simulink model "AC_DC"  (R2022b)
settings: Solver=FixedStepDiscrete  StartTime=0.0  StopTime=2  FixedStep=1e-6  RelTol=1e-3
libraries: spsRMSLib x11, spsSeriesRLCBranchLib x9, simulink x7, spsVoltageMeasurementLib x7, spsCurrentMeasurementLib x6, spsMosfetLib x6, spsIdealSwitchLib x3, spsFourierLib x2, spsMeanLib x2, slpidlib x2, sps_lib x1, spsControlledVoltageSourceLib x1
(part 2 of 2)

== matlab function AC_DC/MATLAB Function22 ==
  data: alpha input; d output; beta input; theta input; q output
function [d, q] = Park_Transform(alpha, beta, theta)
% Park变换模块（直接输入SOGI-FLL的theta，无内部积分）
% 输入：
%   alpha - α轴分量（SOGI-FLL的U_prime）
%   beta  - β轴分量（SOGI-FLL的deltaU_prime）
%   theta - 瞬时相位（SOGI-FLL直接输出的theta）
% 输出：
%   d         - d轴（直轴）分量
%   q         - q轴（交轴）分量
%   cos_theta - 相位θ的余弦值（新增输出）
%   sin_theta - 相位θ的正弦值（新增输出）

%% 核心计算
cos_theta = cos(theta);  % 相位θ的余弦值
sin_theta = sin(theta);  % 相位θ的正弦值


% 修正后的 Park 变换公式（d轴对齐同相分量 beta）
d =  alpha * cos_theta + beta * sin_theta;
q = -alpha * sin_theta + beta * cos_theta;
end

== matlab function AC_DC/MATLAB Function16 ==
  data: in1 input; out1 output; in2 input; in3 input; in4 input; in5 input; in6 input; in7 input; t input; out2 output; out3 output; out4 output; out5 output; out6 output; out7 output
function [out1, out2, out3, out4, out5, out6, out7] = fcn(in1, in2, in3, in4, in5, in6, in7, t)
% 输入：
% in1~in7 : 7路采样信号
% t       : 仿真时间 (需连接Clock模块)
% 输出：
% out1~out7: 0.4秒前全为0，0.4秒后输出采样值

% ====================== 核心判断（只有一行） ======================
if t >= 0.4
    % 时间到：输出采样值
    out1 = in1;
    out2 = in2;
    out3 = in3;
    out4 = in4;
    out5 = in5;
    out6 = in6;
    out7 = in7;
else
    % 时间未到：全部输出0
    out1 = 0;
    out2 = 0;
    out3 = 0;
    out4 = 0;
    out5 = 0;
    out6 = 0;
    out7 = 0;
end

== matlab function AC_DC/MATLAB Function23 ==
  data: I_ref input; duty_out output; I_fb input
function duty_out = fcn(I_ref, I_fb)
%#codegen
% 同步Boost电流环PI控制器（带钳位抗饱和）
% 适配：20kHz采样、±5A电流传感器、占空比0.1~0.9安全范围
% 输入：
%   I_ref: 电压环输出的电流给定（对应你模型里电压环PI的输出）
%   I_fb: 电流反馈（对应你模型里经过-1增益后的IL信号）
% 输出：
%   duty_out: 最终占空比，直接接你模型里的1/z延迟模块

% 持久化变量：保存积分器状态，每个控制周期保留数值
persistent integral_val;
% 初始化：仅仿真启动的第一个控制周期执行1次
if isempty(integral_val)
    integral_val = 0;
end

% ==================== 1. 控制参数（和你原PI模块参数完全一致，可直接修改）====================
Kp = 0.5;       % 比例增益，和你原设置一致
Ki = 10;         % 积分增益，和你原设置一致
Ts = 5e-5;       % 20kHz控制周期，固定不变
% ==================== 2. 物理极限设置（核心抗饱和阈值）====================
DUTY_MAX = 0.93;  % 占空比上限，避免上下管直通
DUTY_MIN = -0.07;  % 占空比下限，杜绝轻载反向电流
I_SAT_LIMIT = 10; % 电流传感器饱和阈值，接近±5A量程提前触发保护

% ==================== 3. 误差计算 ====================
err = I_ref - I_fb;

% ==================== 4. 比例项输出 ====================
prop_out = Kp * err;

% ==================== 5. 核心抗饱和逻辑 ====================
% 5.1 积分项预计算
integral_inc = Ki * Ts * err;
integral_pre = integral_val + integral_inc;
% 5.2 预计算不饱和的PI输出
duty_pre = prop_out + integral_pre;

% 5.3 钳位抗饱和规则：
% 仅当输出在线性区、且电流未达到传感器饱和阈值时，才允许积分累加
% 同时加入反向积分放行规则，避免积分锁死
is_duty_linear = (duty_pre < DUTY_MAX) && (duty_pre > DUTY_MIN);
is_current_unsat = (abs(I_fb) < I_SAT_LIMIT);
is_integral_allow = is_duty_linear && is_current_unsat;
is_reverse_integral = (err > 0 && integral_pre < 0) || (err < 0 && integral_pre > 0);

if is_integral_allow || is_reverse_integral
    integral_val = integral_pre;
end

% ==================== 6. 最终占空比计算 + 硬限幅兜底 ====================
duty_out = prop_out + integral_val;
duty_out = min(max(duty_out, DUTY_MIN), DUTY_MAX);

== matlab function AC_DC/MATLAB Function24 ==
  settings: updateMethod=DISCRETE
  data: uin input; alpha output; beta output
function [alpha, beta] = SOGI_FLL_20kHz(uin)
% 严格对应你的 m 文件：20kHz 双线性 PI-FLL
% 输入：uin   单相电压
% 输出：alpha 同相输出 uα = x2
%      beta  正交输出 uβ = omega0*x3

%% 固定参数（和你的m文件完全一致）
dt = 5e-5;
K  = 1.414;
K1 = 0.25;
gamma_p =30;
gamma_i =500;
w_max = 2*pi*60;
w_min = 2*pi*40;

%% 状态持久化
persistent x1_prev x2_prev x3_prev omega0_prev U_prev integral_f first_run;
if isempty(first_run)
    x1_prev = 0;
    x2_prev = 0;
    x3_prev = 0;
    omega0_prev = 2*pi*50;
    U_prev = uin;
    integral_f = 0;
    first_run = false;
end

%% 1. 当前输入
U_curr = uin;
omega0_prev_local = omega0_prev;

%% 2. 频率预畸变
omega_pre = (2/dt) * tan(omega0_prev_local * dt / 2);

%% 3. 状态矩阵 A, B
A_mat = [
    -K1*omega_pre, -K1*omega_pre, 0;
    -K*omega_pre,  -K*omega_pre,  -omega_pre^2;
    0,              1,              0
];
B_mat = [
    K1*omega_pre;
    K*omega_pre;
    0
];

%% 4. 双线性变换
I_mat = eye(3);
M1 = I_mat - (dt/2)*A_mat;
M2 = I_mat + (dt/2)*A_mat;
U_avg = U_curr + U_prev;

x_prev_vec = [x1_prev; x2_prev; x3_prev];
x_curr_vec = M1 \ (M2 * x_prev_vec + (dt/2)*B_mat * U_avg);

x1_curr = x_curr_vec(1);
x2_curr = x_curr_vec(2);
x3_curr = x_curr_vec(3);

%% 5. PI-FLL 频率环
deltaU = U_curr - x1_curr - x2_curr;
deltaU_prime_val = omega0_prev_local * x3_curr;
epsilon_f = deltaU * deltaU_prime_val;

integral_f = integral_f + epsilon_f * dt;
domega0dt = -gamma_p * epsilon_f - gamma_i * integral_f;
omega0_curr = omega0_prev_local + dt * domega0dt;

% 频率限幅
omega0_curr = max(min(omega0_curr, w_max), w_min);

%% 6. 输出 alpha beta
alpha = x2_curr;
beta  = omega0_curr * x3_curr;

%% 7. 更新状态
x1_prev = x1_curr;
x2_prev = x2_curr;
x3_prev = x3_curr;
omega0_prev = omega0_curr;
U_prev = U_curr;

end

== matlab function AC_DC/MATLAB Function25 ==
  data: u_alpha input; theta output; u_beta input; qerror output
function [theta, qerror] = SRF_PLL(u_alpha, u_beta)
% 同步旋转坐标系锁相环 SRF-PLL
% 【已修改为：纯自适应频率版本 → 和你主循环PLL完全一致】
% 输入：u_alpha, u_beta
% 输出：theta 锁相相位, qerror q分量（趋近0）

    %% ===================== 1. 固定参数 =====================
    Ts = 5e-5;               % 20kHz 采样步长（必须匹配）
    
    % PI参数（和你主循环一致）
    kp_pll = 200;
    ki_pll = 7000;

    %% ===================== 2. 持久变量 =====================
    persistent theta_prev
    persistent integral_pll
    
    if isempty(theta_prev)
        theta_prev = 0;
        integral_pll = 0;
    end

    %% ===================== 3. Park 变换 =====================
    cos_theta = cos(theta_prev);
    sin_theta = sin(theta_prev);
    
    u_d =  u_alpha * cos_theta + u_beta * sin_theta;
    u_q = -u_alpha * sin_theta + u_beta * cos_theta;
    
    qerror = u_q;  % q分量（锁相成功→0）

    %% ===================== 4. PI控制器（我的版本：直接输出ω） =====================
    integral_pll = integral_pll + qerror * Ts;          % 积分
    omega_pll    = kp_pll * qerror + ki_pll * integral_pll; % 直接输出角频率

    %% ===================== 5. 积分生成相位 =====================
    theta = theta_prev + omega_pll * Ts;

    %% ===================== 6. 相位归一化（±π） =====================
    if theta > pi
        theta = theta - 2*pi;
    elseif theta < -pi
        theta = theta + 2*pi;
    end

    %% ===================== 7. 更新状态 =====================
    theta_prev = theta;
end

== matlab function AC_DC/MATLAB Function26 ==
  data: in1 input; in2 input; t input; y output
function y = fcn(in1, in2, t)
% 输入：
% in1：0.4秒 ~ 1.4秒 之间输出的信号
% in2：0.4秒前输出的信号
% t   ：仿真时间 (需连接Clock模块)
% 输出：
% y：三段式输出
%    t < 0.4s    → 输出 in2
%    0.4s ≤ t < 1.4s → 输出 in1
%    t ≥ 1.4s    → 输出 0

% ====================== 核心三段式时间判断 ======================
if t >= 1.4
    % 第三段：1.4秒及以后，强制输出0
    y = in1;
elseif t >= 0.4
    % 第二段：0.4秒到1.4秒之间，输出信号1 (in1)
    y = in1;
else
    % 第一段：0.4秒之前，输出信号2 (in2)
    y = in2;
end

== matlab function AC_DC/MATLAB Function15 ==
  data: IGm_total input; Igm_clean output
function Igm_clean = Notch_100Hz_IGm(IGm_total)
% 100Hz陷波滤波器，放在IGm求和后，滤除二次纹波
% 陷波频率100Hz，带宽6Hz，采样率20kHz
% 输入：IGm_total = IGm1 + IGm2
% 输出：Igm_clean = 滤除100Hz纹波后的纯直流信号

%% 历史变量
persistent x_prev1 x_prev2 y_prev1 y_prev2;

%% 固定参数
Ts = 1/20000;
f0 = 100;          % 陷波频率100Hz
bw = 6;            % 陷波带宽6Hz
w0 = 2*pi*f0;
wb = 2*pi*bw;

%% 双线性变换离散化系数
k = 2/Ts;
a0 = k^2 + wb*k + w0^2;
a1 = 2*(w0^2 - k^2);
a2 = k^2 - wb*k + w0^2;
b0 = k^2 + w0^2;
b1 = 2*(w0^2 - k^2);
b2 = k^2 + w0^2;

%% 归一化
b0 = b0/a0;
b1 = b1/a0;
b2 = b2/a0;
a1 = a1/a0;
a2 = a2/a0;

%% 初始化
if isempty(x_prev1)
    x_prev1 = 0; x_prev2 = 0;
    y_prev1 = 0; y_prev2 = 0;
end

%% 差分方程
Igm_clean = b0*IGm_total + b1*x_prev1 + b2*x_prev2 - a1*y_prev1 - a2*y_prev2;

%% 更新历史变量
x_prev2 = x_prev1;
x_prev1 = IGm_total;
y_prev2 = y_prev1;
y_prev1 = Igm_clean;

end

== matlab function AC_DC/MATLAB Function27 ==
  data: t input; utarget output
function utarget = fcn(t)
% 逻辑：
% 0~0.4s   输出 0
% 0.4~0.7s 从 43 平滑上升到 55（柔和曲线，无冲击）
% 0.7s后   保持 55

START_TIME = 0.4;
END_TIME   = 0.7;
INITIAL_V  = 45;
FINAL_V    = 55;

if t < START_TIME
    utarget = 0;                        % 0~0.4s 输出0
elseif t <= END_TIME
    % 平滑上升：余弦曲线（开始慢、中间快、收尾稳）
    tau = (t - START_TIME) / (END_TIME - START_TIME);
    tau_smooth = 0.5 * (1 - cos(pi * tau));  % 平滑曲线
    utarget = INITIAL_V + (FINAL_V - INITIAL_V) * tau_smooth;
else
    utarget = FINAL_V;                  % 0.7s后保持恒定
end

== matlab function AC_DC/MATLAB Function10 ==
  data: alpha input; d output; beta input; theta input; q output
function [d, q] = Park_Transform(alpha, beta, theta)
% Park变换模块（直接输入SOGI-FLL的theta，无内部积分）
% 输入：
%   alpha - α轴分量（SOGI-FLL的U_prime）
%   beta  - β轴分量（SOGI-FLL的deltaU_prime）
%   theta - 瞬时相位（SOGI-FLL直接输出的theta）
% 输出：
%   d         - d轴（直轴）分量
%   q         - q轴（交轴）分量
%   cos_theta - 相位θ的余弦值（新增输出）
%   sin_theta - 相位θ的正弦值（新增输出）

%% 核心计算
cos_theta = cos(theta);  % 相位θ的余弦值
sin_theta = sin(theta);  % 相位θ的正弦值


% 修正后的 Park 变换公式（d轴对齐同相分量 beta）
d =  alpha * cos_theta + beta * sin_theta;
q = -alpha * sin_theta + beta * cos_theta;
end

== matlab function AC_DC/MATLAB Function19 ==
  settings: updateMethod=DISCRETE
  data: uin input; alpha output; beta output
function [alpha, beta] = SOGI_FLL_20kHz(uin)
% 严格对应你的 m 文件：20kHz 双线性 PI-FLL
% 输入：uin   单相电压
% 输出：alpha 同相输出 uα = x2
%      beta  正交输出 uβ = omega0*x3

%% 固定参数（和你的m文件完全一致）
dt = 5e-5;
K  = 1.414;
K1 = 0.25;
gamma_p =30;
gamma_i =500;
w_max = 2*pi*60;
w_min = 2*pi*40;

%% 状态持久化
persistent x1_prev x2_prev x3_prev omega0_prev U_prev integral_f first_run;
if isempty(first_run)
    x1_prev = 0;
    x2_prev = 0;
    x3_prev = 0;
    omega0_prev = 2*pi*50;
    U_prev = uin;
    integral_f = 0;
    first_run = false;
end

%% 1. 当前输入
U_curr = uin;
omega0_prev_local = omega0_prev;

%% 2. 频率预畸变
omega_pre = (2/dt) * tan(omega0_prev_local * dt / 2);

%% 3. 状态矩阵 A, B
A_mat = [
    -K1*omega_pre, -K1*omega_pre, 0;
    -K*omega_pre,  -K*omega_pre,  -omega_pre^2;
    0,              1,              0
];
B_mat = [
    K1*omega_pre;
    K*omega_pre;
    0
];

%% 4. 双线性变换
I_mat = eye(3);
M1 = I_mat - (dt/2)*A_mat;
M2 = I_mat + (dt/2)*A_mat;
U_avg = U_curr + U_prev;

x_prev_vec = [x1_prev; x2_prev; x3_prev];
x_curr_vec = M1 \ (M2 * x_prev_vec + (dt/2)*B_mat * U_avg);

x1_curr = x_curr_vec(1);
x2_curr = x_curr_vec(2);
x3_curr = x_curr_vec(3);

%% 5. PI-FLL 频率环
deltaU = U_curr - x1_curr - x2_curr;
deltaU_prime_val = omega0_prev_local * x3_curr;
epsilon_f = deltaU * deltaU_prime_val;

integral_f = integral_f + epsilon_f * dt;
domega0dt = -gamma_p * epsilon_f - gamma_i * integral_f;
omega0_curr = omega0_prev_local + dt * domega0dt;

% 频率限幅
omega0_curr = max(min(omega0_curr, w_max), w_min);

%% 6. 输出 alpha beta
alpha = x2_curr;
beta  = omega0_curr * x3_curr;

%% 7. 更新状态
x1_prev = x1_curr;
x2_prev = x2_curr;
x3_prev = x3_curr;
omega0_prev = omega0_curr;
U_prev = U_curr;

end

== matlab function AC_DC/MATLAB Function2 ==
  data: u_alpha input; theta output; u_beta input; qerror output
function [theta, qerror] = SRF_PLL(u_alpha, u_beta)
% 同步旋转坐标系锁相环 SRF-PLL
% 【已修改为：纯自适应频率版本 → 和你主循环PLL完全一致】
% 输入：u_alpha, u_beta
% 输出：theta 锁相相位, qerror q分量（趋近0）

    %% ===================== 1. 固定参数 =====================
    Ts = 5e-5;               % 20kHz 采样步长（必须匹配）
    
    % PI参数（和你主循环一致）
    kp_pll = 200;
    ki_pll = 7000;

    %% ===================== 2. 持久变量 =====================
    persistent theta_prev
    persistent integral_pll
    
    if isempty(theta_prev)
        theta_prev = 0;
        integral_pll = 0;
    end

    %% ===================== 3. Park 变换 =====================
    cos_theta = cos(theta_prev);
    sin_theta = sin(theta_prev);
    
    u_d =  u_alpha * cos_theta + u_beta * sin_theta;
    u_q = -u_alpha * sin_theta + u_beta * cos_theta;
    
    qerror = u_q;  % q分量（锁相成功→0）

    %% ===================== 4. PI控制器（我的版本：直接输出ω） =====================
    integral_pll = integral_pll + qerror * Ts;          % 积分
    omega_pll    = kp_pll * qerror + ki_pll * integral_pll; % 直接输出角频率

    %% ===================== 5. 积分生成相位 =====================
    theta = theta_prev + omega_pll * Ts;

    %% ===================== 6. 相位归一化（±π） =====================
    if theta > pi
        theta = theta - 2*pi;
    elseif theta < -pi
        theta = theta + 2*pi;
    end

    %% ===================== 7. 更新状态 =====================
    theta_prev = theta;
end

== matlab function AC_DC/级联谐波抑制4 ==
  data: u input; y output
function y = Cascade_Notch_Filter(u)
% 级联陷波滤波器：滤除3/5/7次固定频率谐波（150/250/350Hz）
% 输入u：待滤波的标量信号
% 输出y：滤波后的标量信号
% 适配：20kHz采样率（Ts=5e-5），和你的控制环完全对齐

    persistent x3_1 x3_2 x5_1 x5_2 x7_1 x7_2 first_run
    persistent b3_0 b3_1 b3_2 a3_1 a3_2
    persistent b5_0 b5_1 b5_2 a5_1 a5_2
    persistent b7_0 b7_1 b7_2 a7_1 a7_2

    %% ===================== 1. 初始化：仅首次运行 =====================
    if isempty(first_run)
        % --- 固定参数 ---
        Fs = 2e4;          % 采样频率 20kHz
        Ts = 1/Fs;            % 采样周期 5e-5s
        wc = 10;              % 截止角频率 25 rad/s
        
        % 目标谐波频率
        w3 = 2*pi*150;  % 3次谐波 150Hz
        w5 = 2*pi*250;  % 5次谐波 250Hz
        w7 = 2*pi*350;  % 7次谐波 350Hz

        % --- Tustin变换预计算系数 ---
        k = 2/Ts;
        k2 = k*k;

        % --- 3次滤波器系数 ---
        [b3_0, b3_1, b3_2, a3_1, a3_2] = calc_coeff(w3, wc, k, k2);
        % --- 5次滤波器系数 ---
        [b5_0, b5_1, b5_2, a5_1, a5_2] = calc_coeff(w5, wc, k, k2);
        % --- 7次滤波器系数 ---
        [b7_0, b7_1, b7_2, a7_1, a7_2] = calc_coeff(w7, wc, k, k2);

        % --- 显式初始化状态变量为标量 ---
        x3_1 = 0; x3_2 = 0;
        x5_1 = 0; x5_2 = 0;
        x7_1 = 0; x7_2 = 0;
        
        first_run = 1;
    end

    %% ===================== 2. 级联滤波计算（显式差分方程） =====================
    % --- 第1级：3次谐波滤波 ---
    y3 = b3_0*u + x3_1;
    x3_1_next = b3_1*u - a3_1*y3 + x3_2;
    x3_2_next = b3_2*u - a3_2*y3;
    
    % --- 第2级：5次谐波滤波 ---
    y5 = b5_0*y3 + x5_1;
    x5_1_next = b5_1*y3 - a5_1*y5 + x5_2;
    x5_2_next = b5_2*y3 - a5_2*y5;
    
    % --- 第3级：7次谐波滤波 ---
    y7 = b7_0*y5 + x7_1;
    x7_1_next = b7_1*y5 - a7_1*y7 + x7_2;
    x7_2_next = b7_2*y5 - a7_2*y7;
    
    % --- 更新状态变量 ---
    x3_1 = x3_1_next; x3_2 = x3_2_next;
    x5_1 = x5_1_next; x5_2 = x5_2_next;
    x7_1 = x7_1_next; x7_2 = x7_2_next;
    
    % --- 最终输出 ---
    y = y7;

end

%% ===================== 局部函数：预计算滤波器系数 =====================
function [b0, b1, b2, a1, a2] = calc_coeff(wn, wc, k, k2)
    % 连续域：G(s) = (s^2 + wn^2) / (s^2 + 2*wc*s + wn^2)
    % Tustin离散化：s = k*(z-1)/(z+1)
    
    % 连续域系数
    num_b0 = 1; num_b1 = 0; num_b2 = wn^2;
    den_a0 = 1; den_a1 = 2*wc; den_a2 = wn^2;
    
    % 离散化计算
    B0 = num_b0*k2 + num_b1*k + num_b2;
    B1 = 2*num_b2 - 2*num_b0*k2;
    B2 = num_b0*k2 - num_b1*k + num_b2;
    
    A0 = den_a0*k2 + den_a1*k + den_a2;
    A1 = 2*den_a2 - 2*den_a0*k2;
    A2 = den_a0*k2 - den_a1*k + den_a2;
    
    % 归一化（a0=1）
    b0 = B0 / A0;
    b1 = B1 / A0;
    b2 = B2 / A0;
    a1 = A1 / A0;
    a2 = A2 / A0;
end

== matlab function AC_DC/MATLAB Function20 ==
  data: i_error input; m output
function m  = QPR_Current_Loop(i_error)
% 单相LCL整流器 电流环 多谐振QPR控制器
% 【严格匹配论文公式】G = Kp + Σ(2Kr·wi·s)/(s²+2wi·s + wn²)
% 谐振项：基波50Hz + 3次150Hz +5次250Hz +7次350Hz
% 【参数规则】仅Kp全局共用，Kr/wi/w0 每项独立设置
% 采样率：20kHz | 双线性变换离散化

%% ===================== 独立历史变量 =====================
persistent e1_1 e1_2 m1_1 m1_2  % 基波 n=1
persistent e3_1 e3_2 m3_1 m3_2  % 3次  n=3
persistent e5_1 e5_2 m5_1 m5_2  % 5次  n=5
persistent e7_1 e7_2 m7_1 m7_2  % 7次  n=7

%% ===================== 全局共用参数（仅Kp） =====================
Ts    = 1/20000;   % 采样周期
Kp    =0.3;       % 【唯一共用参数】比例增益

%% ===================== 各谐振项 独立参数（互不共用） =====================
% === 基波 50Hz (n=1) ===
Kr1 = 40;
wi1 = 10;
w01 = 100*pi;

% === 3次谐波 150Hz (n=3) ===
Kr3 = 100;
wi3 = 6;
w03 = 300*pi;

% === 5次谐波 250Hz (n=5) ===
Kr5 = 80;
wi5 = 6;
w05 = 500*pi;

% === 7次谐波 350Hz (n=7) ===
Kr7 = 60;
wi7 = 6;
w07 = 700*pi;

%% ===================== 初始化 =====================
if isempty(e1_1)
    e1_1=0;e1_2=0;m1_1=0;m1_2=0;
    e3_1=0;e3_2=0;m3_1=0;m3_2=0;
    e5_1=0;e5_2=0;m5_1=0;m5_2=0;
    e7_1=0;e7_2=0;m7_1=0;m7_2=0;
end

%% ===================== 1. 共用比例项 =====================
m_p = Kp * i_error;

%% ===================== 2. 基波谐振项计算 =====================
A1  = 2 * Kr1 * wi1;
B1  = 2 * wi1;
C1  = w01^2;
a0_1 = 4 + 2*B1*Ts + C1*Ts^2;
a1_1 = -8 + 2*C1*Ts^2;
a2_1 = 4 - 2*B1*Ts + C1*Ts^2;
b0_1 =  A1 * Ts;
b1_1 =  0;
b2_1 = -A1 * Ts;
m1 = (b0_1*i_error + b1_1*e1_1 + b2_1*e1_2 - a1_1*m1_1 - a2_1*m1_2) / a0_1;
% 更新
e1_2 = e1_1; e1_1 = i_error;
m1_2 = m1_1; m1_1 = m1;

%% ===================== 3. 3次谐波谐振项计算 =====================
A3  = 2 * Kr3 * wi3;
B3  = 2 * wi3;
C3  = w03^2;
a0_3 = 4 + 2*B3*Ts + C3*Ts^2;
a1_3 = -8 + 2*C3*Ts^2;
a2_3 = 4 - 2*B3*Ts + C3*Ts^2;
b0_3 =  A3 * Ts;
b1_3 =  0;
b2_3 = -A3 * Ts;
m3 = (b0_3*i_error + b1_3*e3_1 + b2_3*e3_2 - a1_3*m3_1 - a2_3*m3_2) / a0_3;
% 更新
e3_2 = e3_1; e3_1 = i_error;
m3_2 = m3_1; m3_1 = m3;

%% ===================== 4. 5次谐波谐振项计算 =====================
A5  = 2 * Kr5 * wi5;
B5  = 2 * wi5;
C5  = w05^2;
a0_5 = 4 + 2*B5*Ts + C5*Ts^2;
a1_5 = -8 + 2*C5*Ts^2;
a2_5 = 4 - 2*B5*Ts + C5*Ts^2;
b0_5 =  A5 * Ts;
b1_5 =  0;
b2_5 = -A5 * Ts;
m5 = (b0_5*i_error + b1_5*e5_1 + b2_5*e5_2 - a1_5*m5_1 - a2_5*m5_2) / a0_5;
% 更新
e5_2 = e5_1; e5_1 = i_error;
m5_2 = m5_1; m5_1 = m5;

%% ===================== 5. 7次谐波谐振项计算 =====================
A7  = 2 * Kr7 * wi7;
B7  = 2 * wi7;
C7  = w07^2;
a0_7 = 4 + 2*B7*Ts + C7*Ts^2;
a1_7 = -8 + 2*C7*Ts^2;
a2_7 = 4 - 2*B7*Ts + C7*Ts^2;
b0_7 =  A7 * Ts;
b1_7 =  0;
b2_7 = -A7 * Ts;
m7 = (b0_7*i_error + b1_7*e7_1 + b2_7*e7_2 - a1_7*m7_1 - a2_7*m7_2) / a0_7;
% 更新
e7_2 = e7_1; e7_1 = i_error;
m7_2 = m7_1; m7_1 = m7;

%% ===================== 总输出叠加 =====================
m = m_p + m1 + m3 + m5 + m7;



end

== matlab function AC_DC/合闸后再传入信号1 ==
  data: t input; Uref output; Udc input; Udc_error output
function [Uref, Udc_error] = Udc_Control_Logic(t, Udc)
% 单相整流器 直流母线电压 合闸综合控制逻辑
% 功能：
%   1. 0.15s合闸前：Uref=0，不计算误差（Udc_error=0）
%   2. 0.15s后：Uref直接跳变到40V，开始计算误差 Udc_error = 40 - Udc
% 输入：
%   t: 仿真时间
%   Udc: 实际直流母线电压测量值
% 输出：
%   Uref: 直流母线电压给定值
%   Udc_error: 电压误差 = Uref - Udc（合闸后才有值）

persistent V_target t_start;
if isempty(V_target)
    V_target =55;      % 目标电压，直接给50V
    t_start = 0.15;     % 合闸时间
end

%% 核心逻辑：时间分段控制
if t < t_start
    % === 阶段1：合闸前 ===
    Uref = 0;           % 电压给定为0
    Udc_error = 0;      % 不计算误差，避免误动作
else
    % === 阶段2：合闸后 ===
    Uref = V_target;    % 直接跳变到40V恒定
    Udc_error = Uref - Udc; % 立刻开始计算误差，投入闭环
end

end

== matlab function AC_DC/模仿开关控制3 ==
  data: t input; mod_out output; mod_in input
function mod_out = gate_mod_signal(t, mod_in)
% 功能：0.25s前输出0，0.25s后输出原调制波mod_in
% 输入 t: 仿真时间 (Clock模块)
% 输入 mod_in: 原始调制波信号
% 输出 mod_out: 带使能的调制波信号

t_start =0.15; % 合闸时间

if t < t_start
    mod_out = 0;          % 合闸前强制输出0
else
    mod_out = mod_in;      % 合闸后输出原调制波
end
end

== matlab function AC_DC/MATLAB Function28 ==
  data: in1 input; in2 input; t input; y output
function y = fcn(in1, in2, t)
% 输入：
% in1：0.4秒 ~ 1.4秒 之间输出的信号
% in2：0.4秒前输出的信号
% t   ：仿真时间 (需连接Clock模块)
% 输出：
% y：三段式输出
%    t < 0.4s    → 输出 in2
%    0.4s ≤ t < 1.4s → 输出 in1
%    t ≥ 1.4s    → 输出 0

% ====================== 核心三段式时间判断 ======================
if t >= 1.7
    % 第三段：1.4秒及以后，强制输出0
    y = in2;
elseif t >= 0.4
    % 第二段：0.4秒到1.4秒之间，输出信号1 (in1)
    y = in1;
else
    % 第一段：0.4秒之前，输出信号2 (in2)
    y = in1;
end

== matlab function AC_DC/级联谐波抑制2 ==
  data: u input; y output
function y = Cascade_Notch_Filter(u)
% 级联陷波滤波器：滤除3/5/7次固定频率谐波（150/250/350Hz）
% 输入u：待滤波的标量信号
% 输出y：滤波后的标量信号
% 适配：20kHz采样率（Ts=5e-5），和你的控制环完全对齐

    persistent x3_1 x3_2 x5_1 x5_2 x7_1 x7_2 first_run
    persistent b3_0 b3_1 b3_2 a3_1 a3_2
    persistent b5_0 b5_1 b5_2 a5_1 a5_2
    persistent b7_0 b7_1 b7_2 a7_1 a7_2

    %% ===================== 1. 初始化：仅首次运行 =====================
    if isempty(first_run)
        % --- 固定参数 ---
        Fs = 2e4;          % 采样频率 20kHz
        Ts = 1/Fs;            % 采样周期 5e-5s
        wc = 10;              % 截止角频率 25 rad/s
        
        % 目标谐波频率
        w3 = 2*pi*150;  % 3次谐波 150Hz
        w5 = 2*pi*250;  % 5次谐波 250Hz
        w7 = 2*pi*350;  % 7次谐波 350Hz

        % --- Tustin变换预计算系数 ---
        k = 2/Ts;
        k2 = k*k;

        % --- 3次滤波器系数 ---
        [b3_0, b3_1, b3_2, a3_1, a3_2] = calc_coeff(w3, wc, k, k2);
        % --- 5次滤波器系数 ---
        [b5_0, b5_1, b5_2, a5_1, a5_2] = calc_coeff(w5, wc, k, k2);
        % --- 7次滤波器系数 ---
        [b7_0, b7_1, b7_2, a7_1, a7_2] = calc_coeff(w7, wc, k, k2);

        % --- 显式初始化状态变量为标量 ---
        x3_1 = 0; x3_2 = 0;
        x5_1 = 0; x5_2 = 0;
        x7_1 = 0; x7_2 = 0;
        
        first_run = 1;
    end

    %% ===================== 2. 级联滤波计算（显式差分方程） =====================
    % --- 第1级：3次谐波滤波 ---
    y3 = b3_0*u + x3_1;
    x3_1_next = b3_1*u - a3_1*y3 + x3_2;
    x3_2_next = b3_2*u - a3_2*y3;
    
    % --- 第2级：5次谐波滤波 ---
    y5 = b5_0*y3 + x5_1;
    x5_1_next = b5_1*y3 - a5_1*y5 + x5_2;
    x5_2_next = b5_2*y3 - a5_2*y5;
    
    % --- 第3级：7次谐波滤波 ---
    y7 = b7_0*y5 + x7_1;
    x7_1_next = b7_1*y5 - a7_1*y7 + x7_2;
    x7_2_next = b7_2*y5 - a7_2*y7;
    
    % --- 更新状态变量 ---
    x3_1 = x3_1_next; x3_2 = x3_2_next;
    x5_1 = x5_1_next; x5_2 = x5_2_next;
    x7_1 = x7_1_next; x7_2 = x7_2_next;
    
    % --- 最终输出 ---
    y = y7;

end

%% ===================== 局部函数：预计算滤波器系数 =====================
function [b0, b1, b2, a1, a2] = calc_coeff(wn, wc, k, k2)
    % 连续域：G(s) = (s^2 + wn^2) / (s^2 + 2*wc*s + wn^2)
    % Tustin离散化：s = k*(z-1)/(z+1)
    
    % 连续域系数
    num_b0 = 1; num_b1 = 0; num_b2 = wn^2;
    den_a0 = 1; den_a1 = 2*wc; den_a2 = wn^2;
    
    % 离散化计算
    B0 = num_b0*k2 + num_b1*k + num_b2;
    B1 = 2*num_b2 - 2*num_b0*k2;
    B2 = num_b0*k2 - num_b1*k + num_b2;
    
    A0 = den_a0*k2 + den_a1*k + den_a2;
    A1 = 2*den_a2 - 2*den_a0*k2;
    A2 = den_a0*k2 - den_a1*k + den_a2;
    
    % 归一化（a0=1）
    b0 = B0 / A0;
    b1 = B1 / A0;
    b2 = B2 / A0;
    a1 = A1 / A0;
    a2 = A2 / A0;
end

== matlab function AC_DC/MATLAB Function29 ==
  data: i_error input; m output
% function m  = QPR_Current_Loop(i_error, t)
% %#codegen
% % 单相LCL整流器 电流环 多谐振QPR控制器【仅动态调整Kp】
% % 动态Kp规则：
% %   t < 0.4s：Kp=0.3（保持原值，开环前不工作）
% %   0.4s ≤ t < 1.0s：Kp从10线性平滑降到0.3（延长下降时间）
% %   t ≥ 1.0s：Kp=0.3（稳态小Kp，不放大纹波）
% % 其他谐振项计算完全保留你原有的逻辑
% 
% %% ===================== 独立历史变量 =====================
% persistent e1_1 e1_2 m1_1 m1_2  % 基波 n=1
% persistent e3_1 e3_2 m3_1 m3_2  % 3次  n=3
% persistent e5_1 e5_2 m5_1 m5_2  % 5次  n=5
% persistent e7_1 e7_2 m7_1 m7_2  % 7次  n=7
% 
% %% ===================== 全局共用参数 =====================
% Ts    = 1/20000;   % 采样周期
% 
% %% ===================== 各谐振项 独立参数（完全保留你的原值）=====================
% % === 基波 50Hz (n=1) ===
% Kr1 = 40;
% wi1 = 6;
% w01 = 100*pi;
% 
% % === 3次谐波 150Hz (n=3) ===
% Kr3 = 100;
% wi3 = 6;
% w03 = 300*pi;
% 
% % === 5次谐波 250Hz (n=5) ===
% Kr5 = 80;
% wi5 = 6;
% w05 = 500*pi;
% 
% % === 7次谐波 350Hz (n=7) ===
% Kr7 = 60;
% wi7 = 6;
% w07 = 700*pi;
% 
% %% ===================== 初始化 =====================
% if isempty(e1_1)
%     e1_1=0;e1_2=0;m1_1=0;m1_2=0;
%     e3_1=0;e3_2=0;m3_1=0;m3_2=0;
%     e5_1=0;e5_2=0;m5_1=0;m5_2=0;
%     e7_1=0;e7_2=0;m7_1=0;m7_2=0;
% end
% 
% %% ===================== 核心：仅动态调整Kp（平滑曲线版本） =====================
% t_start = 0.4;  % 开环时间
% t_end   = 1;  % 结束时间
% Kp_start = 0.3;  % 起始值
% Kp_end   = 0.3; % 最终稳态值
% 
% if t < t_start
%     Kp = 0.3;
% elseif t >= t_start && t < t_end
%     % 归一化时间 0~1
%     tau = (t - t_start) / (t_end - t_start);
%     % 余弦平滑曲线：开始慢、中间快、结束慢 → 无超调无冲击
%     tau_smooth = 0.5 * (1 - cos(pi * tau));
%     % 计算平滑Kp
%     Kp = Kp_start - (Kp_start - Kp_end) * tau_smooth;
% else
%     Kp = Kp_end;
% end
% %% ===================== 1. 共用比例项（用动态Kp）=====================
% 
% m_p = Kp * i_error;
% 
% %% ===================== 2. 基波谐振项计算（完全保留你的逻辑）=====================
% A1  = 2 * Kr1 * wi1;
% B1  = 2 * wi1;
% C1  = w01^2;
% a0_1 = 4 + 2*B1*Ts + C1*Ts^2;
% a1_1 = -8 + 2*C1*Ts^2;
% a2_1 = 4 - 2*B1*Ts + C1*Ts^2;
% b0_1 =  A1 * Ts;
% b1_1 =  0;
% b2_1 = -A1 * Ts;
% m1 = (b0_1*i_error + b1_1*e1_1 + b2_1*e1_2 - a1_1*m1_1 - a2_1*m1_2) / a0_1;
% % 更新
% e1_2 = e1_1; e1_1 = i_error;
% m1_2 = m1_1; m1_1 = m1;
% 
% %% ===================== 3. 3次谐波谐振项计算（完全保留你的逻辑）=====================
% A3  = 2 * Kr3 * wi3;
% B3  = 2 * wi3;
% C3  = w03^2;
% a0_3 = 4 + 2*B3*Ts + C3*Ts^2;
% a1_3 = -8 + 2*C3*Ts^2;
% a2_3 = 4 - 2*B3*Ts + C3*Ts^2;
% b0_3 =  A3 * Ts;
% b1_3 =  0;
% b2_3 = -A3 * Ts;
% m3 = (b0_3*i_error + b1_3*e3_1 + b2_3*e3_2 - a1_3*m3_1 - a2_3*m3_2) / a0_3;
% % 更新
% e3_2 = e3_1; e3_1 = i_error;
% m3_2 = m3_1; m3_1 = m3;
% 
% %% ===================== 4. 5次谐波谐振项计算（完全保留你的逻辑）=====================
% A5  = 2 * Kr5 * wi5;
% B5  = 2 * wi5;
% C5  = w05^2;
% a0_5 = 4 + 2*B5*Ts + C5*Ts^2;
% a1_5 = -8 + 2*C5*Ts^2;
% a2_5 = 4 - 2*B5*Ts + C5*Ts^2;
% b0_5 =  A5 * Ts;
% b1_5 =  0;
% b2_5 = -A5 * Ts;
% m5 = (b0_5*i_error + b1_5*e5_1 + b2_5*e5_2 - a1_5*m5_1 - a2_5*m5_2) / a0_5;
% % 更新
% e5_2 = e5_1; e5_1 = i_error;
% m5_2 = m5_1; m5_1 = m5;
% 
% %% ===================== 5. 7次谐波谐振项计算（完全保留你的逻辑）=====================
% A7  = 2 * Kr7 * wi7;
% B7  = 2 * wi7;
% C7  = w07^2;
% a0_7 = 4 + 2*B7*Ts + C7*Ts^2;
% a1_7 = -8 + 2*C7*Ts^2;
% a2_7 = 4 - 2*B7*Ts + C7*Ts^2;
% b0_7 =  A7 * Ts;
% b1_7 =  0;
% b2_7 = -A7 * Ts;
% m7 = (b0_7*i_error + b1_7*e7_1 + b2_7*e7_2 - a1_7*m7_1 - a2_7*m7_2) / a0_7;
% % 更新
% e7_2 = e7_1; e7_1 = i_error;
% m7_2 = m7_1; m7_1 = m7;
% 
% %% ===================== 总输出叠加 =====================
% m = m_p + m1 + m3 + m5 + m7;
% 
% end


function m  = QPR_Current_Loop(i_error)
%#codegen
% 单相LCL整流器 电流环 多谐振QPR控制器【固定Kp=0.3 + 频率预畸变】
% 特点：加入双线性变换频率预畸变，保证数字谐振频率准确

%% ===================== 独立历史变量 =====================
persistent e1_1 e1_2 m1_1 m1_2  % 基波 n=1
persistent e3_1 e3_2 m3_1 m3_2  % 3次  n=3
persistent e5_1 e5_2 m5_1 m5_2  % 5次  n=5
persistent e7_1 e7_2 m7_1 m7_2  % 7次  n=7

%% ===================== 全局共用参数 =====================
Ts    = 1/20000;   % 采样周期
Kp    = 0.3;        % 固定比例增益

%% ===================== 各谐振项 独立参数（含频率预畸变）=====================
% === 基波 50Hz (n=1) ===
Kr1 = 40;
wi1 = 6;
f1 = 50;
omega_analog_1 = 2*pi*f1;
w01 = (2/Ts)*tan(omega_analog_1*Ts/2); % 频率预畸变

% === 3次谐波 150Hz (n=3) ===
Kr3 = 100;
wi3 = 6;
f3 = 150;
omega_analog_3 = 2*pi*f3;
w03 = (2/Ts)*tan(omega_analog_3*Ts/2); % 频率预畸变

% === 5次谐波 250Hz (n=5) ===
Kr5 = 80;
wi5 = 6;
f5 = 250;
omega_analog_5 = 2*pi*f5;
w05 = (2/Ts)*tan(omega_analog_5*Ts/2); % 频率预畸变

% === 7次谐波 350Hz (n=7) ===
Kr7 = 60;
wi7 = 6;
f7 = 350;
omega_analog_7 = 2*pi*f7;
w07 = (2/Ts)*tan(omega_analog_7*Ts/2); % 频率预畸变

%% ===================== 初始化 =====================
if isempty(e1_1)
    e1_1=0;e1_2=0;m1_1=0;m1_2=0;
    e3_1=0;e3_2=0;m3_1=0;m3_2=0;
    e5_1=0;e5_2=0;m5_1=0;m5_2=0;
    e7_1=0;e7_2=0;m7_1=0;m7_2=0;
end

%% ===================== 1. 共用比例项（固定Kp）=====================
m_p = Kp * i_error;

%% ===================== 2. 基波谐振项计算 =====================
A1  = 2 * Kr1 * wi1;
B1  = 2 * wi1;
C1  = w01^2;
a0_1 = 4 + 2*B1*Ts + C1*Ts^2;
a1_1 = -8 + 2*C1*Ts^2;
a2_1 = 4 - 2*B1*Ts + C1*Ts^2;
b0_1 =  A1 * Ts;
b1_1 =  0;
b2_1 = -A1 * Ts;
m1 = (b0_1*i_error + b1_1*e1_1 + b2_1*e1_2 - a1_1*m1_1 - a2_1*m1_2) / a0_1;
% 更新
e1_2 = e1_1; e1_1 = i_error;
m1_2 = m1_1; m1_1 = m1;

%% ===================== 3. 3次谐波谐振项计算 =====================
A3  = 2 * Kr3 * wi3;
B3  = 2 * wi3;
C3  = w03^2;
a0_3 = 4 + 2*B3*Ts + C3*Ts^2;
a1_3 = -8 + 2*C3*Ts^2;
a2_3 = 4 - 2*B3*Ts + C3*Ts^2;
b0_3 =  A3 * Ts;
b1_3 =  0;
b2_3 = -A3 * Ts;
m3 = (b0_3*i_error + b1_3*e3_1 + b2_3*e3_2 - a1_3*m3_1 - a2_3*m3_2) / a0_3;
% 更新
e3_2 = e3_1; e3_1 = i_error;
m3_2 = m3_1; m3_1 = m3;

%% ===================== 4. 5次谐波谐振项计算 =====================
A5  = 2 * Kr5 * wi5;
B5  = 2 * wi5;
C5  = w05^2;
a0_5 = 4 + 2*B5*Ts + C5*Ts^2;
a1_5 = -8 + 2*C5*Ts^2;
a2_5 = 4 - 2*B5*Ts + C5*Ts^2;
b0_5 =  A5 * Ts;
b1_5 =  0;
b2_5 = -A5 * Ts;
m5 = (b0_5*i_error + b1_5*e5_1 + b2_5*e5_2 - a1_5*m5_1 - a2_5*m5_2) / a0_5;
% 更新
e5_2 = e5_1; e5_1 = i_error;
m5_2 = m5_1; m5_1 = m5;

%% ===================== 5. 7次谐波谐振项计算 =====================
A7  = 2 * Kr7 * wi7;
B7  = 2 * wi7;
C7  = w07^2;
a0_7 = 4 + 2*B7*Ts + C7*Ts^2;
a1_7 = -8 + 2*C7*Ts^2;
a2_7 = 4 - 2*B7*Ts + C7*Ts^2;
b0_7 =  A7 * Ts;
b1_7 =  0;
b2_7 = -A7 * Ts;
m7 = (b0_7*i_error + b1_7*e7_1 + b2_7*e7_2 - a1_7*m7_1 - a2_7*m7_2) / a0_7;
% 更新
e7_2 = e7_1; e7_1 = i_error;
m7_2 = m7_1; m7_1 = m7;

%% ===================== 总输出叠加 =====================
m = m_p + m1 + m3 + m5 + m7;

end

== matlab function AC_DC/MATLAB Function3 ==
  data: alpha input; d output; beta input; theta input; q output
function [d, q] = Park_Transform(alpha, beta, theta)
% Park变换模块（直接输入SOGI-FLL的theta，无内部积分）
% 输入：
%   alpha - α轴分量（SOGI-FLL的U_prime）
%   beta  - β轴分量（SOGI-FLL的deltaU_prime）
%   theta - 瞬时相位（SOGI-FLL直接输出的theta）
% 输出：
%   d         - d轴（直轴）分量
%   q         - q轴（交轴）分量
%   cos_theta - 相位θ的余弦值（新增输出）
%   sin_theta - 相位θ的正弦值（新增输出）

%% 核心计算
cos_theta = cos(theta);  % 相位θ的余弦值
sin_theta = sin(theta);  % 相位θ的正弦值


% 修正后的 Park 变换公式（d轴对齐同相分量 beta）
d =  alpha * cos_theta + beta * sin_theta;
q = -alpha * sin_theta + beta * cos_theta;
end

== matlab function AC_DC/MATLAB Function4 ==
  data: I_ref input; duty_out output; I_fb input
function duty_out = fcn(I_ref, I_fb)
%#codegen
% 同步Boost电流环PI控制器（带钳位抗饱和）
% 适配：20kHz采样、±5A电流传感器、占空比0.1~0.9安全范围
% 输入：
%   I_ref: 电压环输出的电流给定（对应你模型里电压环PI的输出）
%   I_fb: 电流反馈（对应你模型里经过-1增益后的IL信号）
% 输出：
%   duty_out: 最终占空比，直接接你模型里的1/z延迟模块

% 持久化变量：保存积分器状态，每个控制周期保留数值
persistent integral_val;
% 初始化：仅仿真启动的第一个控制周期执行1次
if isempty(integral_val)
    integral_val = 0;
end

% ==================== 1. 控制参数（和你原PI模块参数完全一致，可直接修改）====================
Kp = 0.5;       % 比例增益，和你原设置一致
Ki = 10;         % 积分增益，和你原设置一致
Ts = 5e-5;       % 20kHz控制周期，固定不变
% ==================== 2. 物理极限设置（核心抗饱和阈值）====================
DUTY_MAX = 0.93;  % 占空比上限，避免上下管直通
DUTY_MIN = -0.07;  % 占空比下限，杜绝轻载反向电流
I_SAT_LIMIT = 10; % 电流传感器饱和阈值，接近±5A量程提前触发保护

% ==================== 3. 误差计算 ====================
err = I_ref - I_fb;

% ==================== 4. 比例项输出 ====================
prop_out = Kp * err;

% ==================== 5. 核心抗饱和逻辑 ====================
% 5.1 积分项预计算
integral_inc = Ki * Ts * err;
integral_pre = integral_val + integral_inc;
% 5.2 预计算不饱和的PI输出
duty_pre = prop_out + integral_pre;

% 5.3 钳位抗饱和规则：
% 仅当输出在线性区、且电流未达到传感器饱和阈值时，才允许积分累加
% 同时加入反向积分放行规则，避免积分锁死
is_duty_linear = (duty_pre < DUTY_MAX) && (duty_pre > DUTY_MIN);
is_current_unsat = (abs(I_fb) < I_SAT_LIMIT);
is_integral_allow = is_duty_linear && is_current_unsat;
is_reverse_integral = (err > 0 && integral_pre < 0) || (err < 0 && integral_pre > 0);

if is_integral_allow || is_reverse_integral
    integral_val = integral_pre;
end

% ==================== 6. 最终占空比计算 + 硬限幅兜底 ====================
duty_out = prop_out + integral_val;
duty_out = min(max(duty_out, DUTY_MIN), DUTY_MAX);

== matlab function AC_DC/MATLAB Function5 ==
  settings: updateMethod=DISCRETE
  data: uin input; alpha output; beta output
function [alpha, beta] = SOGI_FLL_20kHz(uin)
% 严格对应你的 m 文件：20kHz 双线性 PI-FLL
% 输入：uin   单相电压
% 输出：alpha 同相输出 uα = x2
%      beta  正交输出 uβ = omega0*x3

%% 固定参数（和你的m文件完全一致）
dt = 5e-5;
K  = 1.414;
K1 = 0.25;
gamma_p =30;
gamma_i =500;
w_max = 2*pi*60;
w_min = 2*pi*40;

%% 状态持久化
persistent x1_prev x2_prev x3_prev omega0_prev U_prev integral_f first_run;
if isempty(first_run)
    x1_prev = 0;
    x2_prev = 0;
    x3_prev = 0;
    omega0_prev = 2*pi*50;
    U_prev = uin;
    integral_f = 0;
    first_run = false;
end

%% 1. 当前输入
U_curr = uin;
omega0_prev_local = omega0_prev;

%% 2. 频率预畸变
omega_pre = (2/dt) * tan(omega0_prev_local * dt / 2);

%% 3. 状态矩阵 A, B
A_mat = [
    -K1*omega_pre, -K1*omega_pre, 0;
    -K*omega_pre,  -K*omega_pre,  -omega_pre^2;
    0,              1,              0
];
B_mat = [
    K1*omega_pre;
    K*omega_pre;
    0
];

%% 4. 双线性变换
I_mat = eye(3);
M1 = I_mat - (dt/2)*A_mat;
M2 = I_mat + (dt/2)*A_mat;
U_avg = U_curr + U_prev;

x_prev_vec = [x1_prev; x2_prev; x3_prev];
x_curr_vec = M1 \ (M2 * x_prev_vec + (dt/2)*B_mat * U_avg);

x1_curr = x_curr_vec(1);
x2_curr = x_curr_vec(2);
x3_curr = x_curr_vec(3);

%% 5. PI-FLL 频率环
deltaU = U_curr - x1_curr - x2_curr;
deltaU_prime_val = omega0_prev_local * x3_curr;
epsilon_f = deltaU * deltaU_prime_val;

integral_f = integral_f + epsilon_f * dt;
domega0dt = -gamma_p * epsilon_f - gamma_i * integral_f;
omega0_curr = omega0_prev_local + dt * domega0dt;

% 频率限幅
omega0_curr = max(min(omega0_curr, w_max), w_min);

%% 6. 输出 alpha beta
alpha = x2_curr;
beta  = omega0_curr * x3_curr;

%% 7. 更新状态
x1_prev = x1_curr;
x2_prev = x2_curr;
x3_prev = x3_curr;
omega0_prev = omega0_curr;
U_prev = U_curr;

end

== matlab function AC_DC/MATLAB Function6 ==
  data: u_alpha input; theta output; u_beta input; qerror output
function [theta, qerror] = SRF_PLL(u_alpha, u_beta)
% 同步旋转坐标系锁相环 SRF-PLL
% 【已修改为：纯自适应频率版本 → 和你主循环PLL完全一致】
% 输入：u_alpha, u_beta
% 输出：theta 锁相相位, qerror q分量（趋近0）

    %% ===================== 1. 固定参数 =====================
    Ts = 5e-5;               % 20kHz 采样步长（必须匹配）
    
    % PI参数（和你主循环一致）
    kp_pll = 200;
    ki_pll = 7000;

    %% ===================== 2. 持久变量 =====================
    persistent theta_prev
    persistent integral_pll
    
    if isempty(theta_prev)
        theta_prev = 0;
        integral_pll = 0;
    end

    %% ===================== 3. Park 变换 =====================
    cos_theta = cos(theta_prev);
    sin_theta = sin(theta_prev);
    
    u_d =  u_alpha * cos_theta + u_beta * sin_theta;
    u_q = -u_alpha * sin_theta + u_beta * cos_theta;
    
    qerror = u_q;  % q分量（锁相成功→0）

    %% ===================== 4. PI控制器（我的版本：直接输出ω） =====================
    integral_pll = integral_pll + qerror * Ts;          % 积分
    omega_pll    = kp_pll * qerror + ki_pll * integral_pll; % 直接输出角频率

    %% ===================== 5. 积分生成相位 =====================
    theta = theta_prev + omega_pll * Ts;

    %% ===================== 6. 相位归一化（±π） =====================
    if theta > pi
        theta = theta - 2*pi;
    elseif theta < -pi
        theta = theta + 2*pi;
    end

    %% ===================== 7. 更新状态 =====================
    theta_prev = theta;
end

== matlab function AC_DC/MATLAB Function7 ==
  data: in1 input; in2 input; t input; y output
function y = fcn(in1, in2, t)
% 输入：
% in1：0.4秒 ~ 1.4秒 之间输出的信号
% in2：0.4秒前输出的信号
% t   ：仿真时间 (需连接Clock模块)
% 输出：
% y：三段式输出
%    t < 0.4s    → 输出 in2
%    0.4s ≤ t < 1.4s → 输出 in1
%    t ≥ 1.4s    → 输出 0

% ====================== 核心三段式时间判断 ======================
if t >= 1.4
    % 第三段：1.4秒及以后，强制输出0
    y = in1;
elseif t >= 0.4
    % 第二段：0.4秒到1.4秒之间，输出信号1 (in1)
    y = in1;
else
    % 第一段：0.4秒之前，输出信号2 (in2)
    y = in2;
end

== matlab function AC_DC/MATLAB Function8 ==
  data: t input; utarget output
function utarget = fcn(t)
% 逻辑：
% 0~0.4s   输出 0
% 0.4~0.7s 从 43 平滑上升到 55（柔和曲线，无冲击）
% 0.7s后   保持 55

START_TIME = 0.4;
END_TIME   = 0.7;
INITIAL_V  = 45;
FINAL_V    = 55;

if t < START_TIME
    utarget = 0;                        % 0~0.4s 输出0
elseif t <= END_TIME
    % 平滑上升：余弦曲线（开始慢、中间快、收尾稳）
    tau = (t - START_TIME) / (END_TIME - START_TIME);
    tau_smooth = 0.5 * (1 - cos(pi * tau));  % 平滑曲线
    utarget = INITIAL_V + (FINAL_V - INITIAL_V) * tau_smooth;
else
    utarget = FINAL_V;                  % 0.7s后保持恒定
end

== matlab function AC_DC/级联谐波抑制1 ==
  data: u input; y output
function y = Cascade_Notch_Filter(u)
% 级联陷波滤波器：滤除3/5/7次固定频率谐波（150/250/350Hz）
% 输入u：待滤波的标量信号
% 输出y：滤波后的标量信号
% 适配：20kHz采样率（Ts=5e-5），和你的控制环完全对齐

    persistent x3_1 x3_2 x5_1 x5_2 x7_1 x7_2 first_run
    persistent b3_0 b3_1 b3_2 a3_1 a3_2
    persistent b5_0 b5_1 b5_2 a5_1 a5_2
    persistent b7_0 b7_1 b7_2 a7_1 a7_2

    %% ===================== 1. 初始化：仅首次运行 =====================
    if isempty(first_run)
        % --- 固定参数 ---
        Fs = 2e4;          % 采样频率 20kHz
        Ts = 1/Fs;            % 采样周期 5e-5s
        wc = 10;              % 截止角频率 25 rad/s
        
        % 目标谐波频率
        w3 = 2*pi*150;  % 3次谐波 150Hz
        w5 = 2*pi*250;  % 5次谐波 250Hz
        w7 = 2*pi*350;  % 7次谐波 350Hz

        % --- Tustin变换预计算系数 ---
        k = 2/Ts;
        k2 = k*k;

        % --- 3次滤波器系数 ---
        [b3_0, b3_1, b3_2, a3_1, a3_2] = calc_coeff(w3, wc, k, k2);
        % --- 5次滤波器系数 ---
        [b5_0, b5_1, b5_2, a5_1, a5_2] = calc_coeff(w5, wc, k, k2);
        % --- 7次滤波器系数 ---
        [b7_0, b7_1, b7_2, a7_1, a7_2] = calc_coeff(w7, wc, k, k2);

        % --- 显式初始化状态变量为标量 ---
        x3_1 = 0; x3_2 = 0;
        x5_1 = 0; x5_2 = 0;
        x7_1 = 0; x7_2 = 0;
        
        first_run = 1;
    end

    %% ===================== 2. 级联滤波计算（显式差分方程） =====================
    % --- 第1级：3次谐波滤波 ---
    y3 = b3_0*u + x3_1;
    x3_1_next = b3_1*u - a3_1*y3 + x3_2;
    x3_2_next = b3_2*u - a3_2*y3;
    
    % --- 第2级：5次谐波滤波 ---
    y5 = b5_0*y3 + x5_1;
    x5_1_next = b5_1*y3 - a5_1*y5 + x5_2;
    x5_2_next = b5_2*y3 - a5_2*y5;
    
    % --- 第3级：7次谐波滤波 ---
    y7 = b7_0*y5 + x7_1;
    x7_1_next = b7_1*y5 - a7_1*y7 + x7_2;
    x7_2_next = b7_2*y5 - a7_2*y7;
    
    % --- 更新状态变量 ---
    x3_1 = x3_1_next; x3_2 = x3_2_next;
    x5_1 = x5_1_next; x5_2 = x5_2_next;
    x7_1 = x7_1_next; x7_2 = x7_2_next;
    
    % --- 最终输出 ---
    y = y7;

end

%% ===================== 局部函数：预计算滤波器系数 =====================
function [b0, b1, b2, a1, a2] = calc_coeff(wn, wc, k, k2)
    % 连续域：G(s) = (s^2 + wn^2) / (s^2 + 2*wc*s + wn^2)
    % Tustin离散化：s = k*(z-1)/(z+1)
    
    % 连续域系数
    num_b0 = 1; num_b1 = 0; num_b2 = wn^2;
    den_a0 = 1; den_a1 = 2*wc; den_a2 = wn^2;
    
    % 离散化计算
    B0 = num_b0*k2 + num_b1*k + num_b2;
    B1 = 2*num_b2 - 2*num_b0*k2;
    B2 = num_b0*k2 - num_b1*k + num_b2;
    
    A0 = den_a0*k2 + den_a1*k + den_a2;
    A1 = 2*den_a2 - 2*den_a0*k2;
    A2 = den_a0*k2 - den_a1*k + den_a2;
    
    % 归一化（a0=1）
    b0 = B0 / A0;
    b1 = B1 / A0;
    b2 = B2 / A0;
    a1 = A1 / A0;
    a2 = A2 / A0;
end

== matlab function AC_DC/MATLAB Function9 ==
  data: in1 input; in2 input; t input; y output
function y = fcn(in1, in2, t)
% 输入：
% in1：0.4秒 ~ 1.4秒 之间输出的信号
% in2：0.4秒前输出的信号
% t   ：仿真时间 (需连接Clock模块)
% 输出：
% y：三段式输出
%    t < 0.4s    → 输出 in2
%    0.4s ≤ t < 1.4s → 输出 in1
%    t ≥ 1.4s    → 输出 0

% ====================== 核心三段式时间判断 ======================
if t >= 1.7
    % 第三段：1.4秒及以后，强制输出0
    y = in2;
elseif t >= 0.4
    % 第二段：0.4秒到1.4秒之间，输出信号1 (in1)
    y = in1;
else
    % 第一段：0.4秒之前，输出信号2 (in2)
    y = in1;
end
